simulink model "q_5dof_wand_vr_sphere_collision_atia"  (Simulink 9.1)
settings: Solver=ode1  StartTime=0.0  StopTime=inf  FixedStep=0.001  RelTol=1e-3  EnableMultiTasking=on
values from neighbouring files (symbols this model uses):
  COM = zeros(1,size(V1,2))    [atia_centroid.m]
  fromSI = [1e3 1e3 1e3 180/pi 180/pi]    [setup_wand.m]
  K_CURR = 0.5 * [1 1 -1 -1 1 1]    [setup_wand.m]
  kd = [kd_x kd_y kd_z kd_yaw kd_roll]    [setup_wand.m]
  kp = [kp_x kp_y kp_z kp_yaw kp_roll]    [setup_wand.m]
  vo_c = [0 75 -75] * 1e-3    [setup_wand.m]
  wn_f = 150    [setup_wand.m]
  zeta_f = 1    [setup_wand.m]
undefined symbols (not defined in the file or in its folder): DiscIntNeverNeededParam, HIL, qc_get_step_size, V_CUBE_atia_wand, Visualization
libraries: quarc_library x12
(part 2 of 2)

== matlab function Virtual Cube/Virtual Cube ==
  data: dir_atia output double; center input double; COM input double; V_CUBE_atia_wand input double; k_stiff input double; k_damp input double; w_xyz input double; F output double; w_dot input double; collisionFlag output double; dist output double; F_ATIA output double
% Inputs:
% center    = center of object (m)
% radius    = radius of object (m)
% k_stiff   = Stiffness gain (N/m)
% k_damp    = Damping gain (N.s/m)
% w         = world coordinates of wand (m,rad)
% w_dot     = world rate of wand (m/s,rad/s)
%
% Output: 
% F = Output force (N)
%radius==V_CUBE_atia_wand
function [dir_atia,F,collisionFlag,dist,F_ATIA]  = virtual_object(center,COM,V_CUBE_atia_wand, k_stiff, k_damp, w_xyz, w_dot)
%%%%%%%%%%%%%%%%%%%%%%%%%%%%%%%%%%%%%%%%%%%%%%%%%%%%%%

scale=1;
position=COM;
%[V_CUBE_atia_wand,COM]=atia_shape_vertecise(scale,V_CUBE_atia_wand,center)
% Example script for GJK function
%   Animates two objects on a collision course and terminates animation
%   when they hit each other. Loads vertex and face data from
%   SampleShapeData.m. See the comments of GJK.m for more information
%
%   Most of this script just sets up the animation and transformations of
%   the shapes. The only key line is:
%   collisionFlag = GJK(S1Obj,S2Obj,iterationsAllowed)
%
%   Matthew Sheen, 2016
%
%
%%%%%%%%%%%%%%%%%%%%% MODIFICTATION NOTICE: %%%%%%%%%%%%%%%%%%%%%%%%%%%%%%%
% This script test has been modified and renamed by PHILIPPE LEBEL 
% April 2017
%
% The author of the original script is Matthew Sheen
% published on
% https://www.mathworks.com/matlabcentral/fileexchange/57907-fast-3d-collision-detection-gjk-algorithm
% 
%
%I (Philippe Lebel) modified it to accommodate tests for my implmenetation of GJK distance
%algorithm. The commented section at the end of the code allows to see the
%minkowski difference and the verticies member of the simplex evolving
%durring the simulation.
%
%The function I wrote is [dist,pts,G,H]=GJK_dist(S1Obj,S2Obj);
% I only take credit for this function.
% I also modified some sections of the other matlab files to accommodate my
% new function.
% I want to personnally thank Matthew Sheen for his work. This allowed me
% to understand a lot concerning the implementation of such algorithm.
%
% The algorithm works in the vast majority of cases, but some times, in
% close proximity, the closest distance points are a little off. There is
% work to be done concerning this bug. Feel free to contribute if you find
% something.




%clc;clear all;close all% khodm % krdm

%How many iterations to allow for collision detection.
iterationsAllowed = 6;

% Make a figure
%fig=figure('units','normalized','outerposition',[0 0 1 1]);
%set(fig, 'renderer', 'OpenGL');

% fig = figure;
%hold on

% Load sample vertex and face data for two convex polyhedra
% SampleShapeData;
%[V1,F1]=platonic_solid(1,1);
% I make a cube here with  0.05, and transfer com of that to center of
% yellow cube

%[V_CUBE_atia_wand,F1]=platonic_solid(2,0.05);
%COM=atia_centroid(V_CUBE_atia_wand);
%diff_atia=[0 0 -0.075]-COM;
 %V_CUBE_atia_wand=V_CUBE_atia_wand+diff_atia;
 %COM=atia_centroid(V_CUBE_atia_wand);%cube center
 
%[V2,F2]=platonic_solid(3,1); put a point instead of a tethrahedron
 V2=[0 0 0];
 F2=[1 1 1];
 
% V_CUBE_atia_wand =([ 0.1000  120.0000  -34.9000
 %        0  120.0000  -35.0000
  %  0.1000  120.0000  -35.0000
   %      0  120.0000  -34.9000
    %0.1000  120.1000  -34.9000
     %    0  120.1000  -34.9000
    %0.1000  120.1000  -35.0000
     %    0  120.1000  -35.0000]*0.001)+([0 210 -225]*0.001)+[0 0 0.035];%cube went tp the wand location
 
  V_CUBE_atia=[  100.0000         0  100.0000
         0         0         0
  100.0000         0         0
       0         0  100.0000
100.0000  100.0000  100.0000
        0  100.0000  100.0000
 100.0000  100.0000         0
        0  100.0000         0];
     V_CUBE_atia= V_CUBE_atia*0.001;
% Make shape 1

%coder.extrinsic('patch'); 
%S1.Vertices = V1;
%S1.Faces = F1;
%S1.FaceVertexCData=0;
%S1.FaceVertexCData = jet(size(V1,1));
% S1.FaceColor='white';
%S1.FaceColor = 'interp';
%S1Obj = patch(S1);
%COM=atia_centroid(V1);
%COM=atia_centroid(V_CUBE_atia_wand);
% Make shape 2

%S2.Vertices = V2;% handle nist 
%%S2.FaceVertexCData=0;
%S2.FaceVertexCData = jet(size(V2,1));
% S2.FaceColor='white';
%S2.FaceColor = 'interp';
%S2Obj = patch(S2);%handle

 %atia_void_figure()
%hold off
%axis equal
%axis([-5 5 -5 5 -5 5])
%fig.Children.Visible = 'off'; % Turn off the axis for more pleasant viewing.
%Color=[1 1 1];
%fig.Color = Color;
%rotate3d on;

%S1Obj.Vertices=zeros(20,3);
%S2Obj.Vertices=zeros(1,3);

%Move them through space arbitrarily.
% I have to replace every S1Obj.Vertices with V1
%S1Obj.Vertices=V1;
%S2Obj.Vertices=V2;
%S1Obj=atia_produce_handle(V1,F1);
%S1Coords = S1Obj.Vertices;
%[S2Obj]=atia_produce_handle(V2,F2);
%S2Coords = S2Obj.Vertices;
%S1Coords =V1;
%S2Coords = V2;

%S1Rot = eye(3,3); % Accumulate angle changes

% Make a random rotation matix to rotate shape 1 by every step
%S1Angs = 0.1*rand(3,1); % Euler angles
% S1Angs=[0 0 0.1]';
%sang1 = sin(S1Angs);
%cang1 = cos(S1Angs);
%cx = cang1(1); cy = cang1(2); cz = cang1(3);
%sx = sang1(1); sy = sang1(2);  sz = sang1(3);

%S1RotDiff = ...
 %   [          cy*cz,          cy*sz,            -sy
%    sy*cx*cz+sz*sx, sy*cx*sz-cz*sx,          cy*cx];

%S2Rot = eye(3,3);

% Make a random rotation matix to rotate shape 2 by every step
%S2Angs = 0.1*rand(3,1); % Euler angles
% S2Angs=[0 0 0]';
%sang2 = sin(S2Angs);
%cang2 = cos(S2Angs);
%cx = cang2(1); cy = cang2(2); cz = cang2(3);
%sx = sang2(1); sy = sang2(2); sz = sang2(3);

%S2RotDiff = ...
%    [          cy*cz,          cy*sz,            -sy
%    sy*sx*cz-sz*cx, sy*sx*sz+cz*cx,          cy*sx
%    sy*cx*cz+sz*sx, sy*cx*sz-cz*sx,          cy*cx];

%%%%%%%%%%%%%%%%%%%%%%%%%%%%%%%%%%%%%%%%%%%%%%%%%%%%%%%%%%%%%%%%%%%%%
%%%%%%%%%%%%%%%%%%%%%%%%%%%%%%%%%%%%%%%%%%%%%%%%%%%%%%%%%%%%%%%%%%%%


% Animation loop. Terminates on collision.
%n=1;
%dist=-1000;
%for i = 2:-0.005:-inf;
%     if n==60
%         break
%     end


%    S1Rot = S1RotDiff*S1Rot;
%    S2Rot = S2RotDiff*S2Rot;
    %S2Rot = [0.0580    0.9510    0.3037];
    
    %S1Obj.Vertices = (S1Rot*S1Coords')' ;
    %S2Obj.Vertices=w_xyz;
%    V1 = (S1Rot*S1Coords')' ;
%    V2=(w_xyz)';
    %S2Obj.Vertices = (S2Rot*S2Coords')'+-i;%point w_xyz
  
    %[S,D]=minksum(V1,-V2);
   % stock.s{n}=S;
   % stock.s1{n}=S1Obj;
   % stock.s2{n}=S2Obj;
    % Do collision detection
   %collisionFlag = GJK(V_CUBE_atia_wand,(w_xyz'),iterationsAllowed);
    %collisionFlag = GJK(S1Obj,S2Obj,iterationsAllowed);
    %[dist,pts,G,H] = GJK_dist( V_CUBE_atia_wand, (w_xyz') )
     %collisionFlag = GJK_mod(V_CUBE_atia_wand,(w_xyz)',iterationsAllowed);
  [a,b,c,d,collisionFlag] = GJK_mod(V_CUBE_atia_wand,(w_xyz'),iterationsAllowed);
    
    %coder.extrinsic('tic');
    %[dist,pts,G,H]=GJK_dist(V1,V2);
    [dist,pts,G,H]=GJK_dist(V_CUBE_atia_wand,(w_xyz)');
    radius_atia=norm(G-(COM));%radius of cube
    r_atia=w_xyz-(COM);
    r_abs_atia=norm(r_atia);
    %coder.extrinsic('toc');
%     stock.pts{n}=pts;
    %try delete(hhh)
    %end
    %hold on
    %plot3(G(1),G(2),G(3),'Ob','Linewidth',3);
    %hold on
   % plot3(H(1),H(2),H(3),'Ob','Linewidth',3);
    %hold on
   %line([G(1) H(1)],[G(2) H(2)],[G(3) H(3)]);
%     [a,b, c,dist]=EPA(a,b,c,d);
    %stock.pts{n}=pts;
    %dist_acc(n)=dist;
%     [q,r]=max(abs(diff(dist_acc)))
%     if max(abs(diff(dist_acc)))>0.1
%         break
%     end
    %n=n+1;
    %drawnow;
    %hold on
    %figure
    dir_atia = (r_atia) / norm((r_atia));
    %plot(collisionFlag(n))
    if collisionFlag
     %if (r_abs_atia<=radius_atia) very ineffective
       % t = text(3,3,3,'Collision!','FontSize',30);
       %  break;
          %dir=w_xyz-(COM)';
         %dir_atia = (r_atia) / norm((r_atia));
         %F_stiff = [dir_atia * k_stiff(1)*100000000000000 *(radius_atia-r_abs_atia); 0; 0];
         %10000000000000000000000 
         F_stiff = [dir_atia * k_stiff(1)* dist; 0; 0];
           %F_stiff = [dir * k_stiff(1)*1000 * norm(w_xyz-(COM)'); 0; 0];
            %F_stiff = [dir * k_stiff(1) * collisionFlag ; 0; 0];
            
    %F_stiff = [dir * k_stiff(1) * (radius - norm(r)); 0; 0];% r_abs replaced by norm(r)
    % damping force (N)
    %100000000000000
    F_damp = - k_damp .* w_dot;
    % total force
    F = F_stiff + F_damp;
    % = F_stiff;
    F_ATIA=F(1:3,1) ;  
    else
         %t = text(3,3,3,' No Collision!','FontSize',30);
         F = [ 0; 0; 0; 0; 0 ];
         F_ATIA=F(1:3,1) ;
    %end
     %drawnow;
    end
%hold on
%figure
%plot(w_xyz(n))
%disp('w_xyz(n)')
%hold on
%dist_acc(end)
% figure
% view(3)
% for i=1:3:length(stock.s)
%     a=stock.s{i};
%     pts=stock.pts{i};
%     pt_x=a(:,1);
%     pt_y=a(:,2);
%     pt_z=a(:,3);
%     T = delaunay(pt_x,pt_y,pt_z);
%     X=[pt_x,pt_y,pt_z];
%     try delete(h1)
%     end
%     try delete(h2)
%     end
%     h1=tetramesh(T,X,'faceColor','b','EdgeColor',[0 0 0],'FaceAlpha',0.1);
%     hold on
%     for j=1:3
%         h2(j)=plot3(pts(1,j),pts(2,j),pts(3,j),'Or','LineWidth',3);
%         hold on
%         d=cross(pts(:,2)-pts(:,1),pts(:,3)-pts(:,1));
%         if d'*pts(:,1)>0
%             d=-d;
%         end
%         line([pts(1,1) pts(1,1)+d(1)],[pts(2,1) pts(2,1)+d(2)],[pts(3,1) pts(3,1)+d(3)])
%         hold on
%     end
%     hold off
%     
%     axis([-1 10 -1 10 -1 10]);
%     drawnow;
%     pause(0.05)
% end
% hold on%%%%%%%%%%%%%%%%%%%%%%%%%

% Vector from object to wand (m)
r = w_xyz - center;
% Distance of r (m)
r_abs = norm( r );
% Is wand inside object?
%if ( (norm(r(1)) < radius) && (norm(r(2)) < radius) && (norm(r(3)) < radius)&& (norm(r)>radius)&&(norm(r)<1.73*radius))
%if((r_abs<radius) )  
% normalized direction vector
    dir = r / norm(r); % r_abs replaced by norm(r)   
    % stiffness force (N)
     %F_stiff = [dir * k_stiff(1) * (radius-r_abs); 0; 0];
    %F_stiff = [dir * k_stiff(1) * (radius - norm(r)); 0; 0];% r_abs replaced by norm(r)
    % damping force (N)
   % F_damp = - k_damp .* w_dot;
    % total force
   % F = F_stiff + F_damp ;
%else
    % Want not touching object.
   % F = [ 0; 0; 0; 0; 0 ];
end

function [V_CUBE_atia_wand,COM]=atia_shape_vertecise(scale,V_CUBE_atia_wand,center)
%[V_CUBE_atia_wand,F]=platonic_solid(n,r);
V_CUBE_atia_wand=V_CUBE_atia_wand*scale;
COM=atia_centroid(V_CUBE_atia_wand);
diff_atia=center'-COM;
 V_CUBE_atia_wand=V_CUBE_atia_wand+diff_atia;
 COM=atia_centroid(V_CUBE_atia_wand);%cube center
end

function COM=atia_centroid(V1)%
% this function take a matris V1 as input, find average for each column,
% and give you mean or center of mass
COM=zeros(1,size(V1,2));
for j=1:size(V1,2)
s1=0;
for i=1:size(V1,1)%20-7
  %  s1=s1+ eval(sprintf('V1%d(i,1)',j));% adds up X value for all columns%p-V1
    % s1=s1+ eval(V1(sprintf('%d',i),j));
      s1=s1+ V1(i,j);
end
COM(1,j)=s1/size(V1,1);%20-7
end
end


%This function is based on the book Real-Time Collision Detection
% (http://realtimecollisiondetection.net/)
%
%It computes the distance, the points of closest proximity points and also
%returns the points last contained in the simplex.
%[dist,pts,G,H] = GJK_dist_7_point_poly( shape1, shape2 )
%
% INPUTS:
%
% shape1:   a patch object representing the first convex solid
% shape2:   a patch object representing the second convex solid
%
% OUTPUTS:
%
% dist:     an absolute float number representing the minimum distance between
%           the shapes.
% pts:      The points of the minkowsky diference where the alogrithm
%           stoped.
% G:        The point on shape1 closest to shape2
% H:        The point on shape2 closest to shape1


% updated 05/01/17. Thanks to Amin Ramezanifar for pointing out an error.


function [dist,pts,G,H] = GJK_dist( shape1, shape2 )

%pick a random direction
d=[1 1 1];
%pick a point
[a, point1_a, point2_a]=support_2(shape1,shape2,d);
%pick a second point to creat a line
[b, point1_b, point2_b]=support_2(shape1,shape2,-d);
%pick a third point to make a tirangle
ab=b-a;
ao=-a;
%perpendicular direction
d=cross(cross(ab,ao),ab);
%pick a third point
[c, point1_c, point2_c]=support_2(shape1,shape2,d);
%the simplex is now complete
pts=[a b c];
pts_1_2=[point1_a point1_b point1_c;point2_a point2_b point2_c];


itt=0;
pts_old=pts;
norm_old=norm(pts_old);
d_old=d;
dist_old=1000;
dist=1000;
flag=0;
%PP0 = 'V';
PP0 = [3 4 12];
%This loop is there for the very rare case where the simplex would contain
%duplicate points.
while true
    if isequal(c,b) || isequal(c,a)
        [c, point1_c, point2_c]=support_2(shape1,shape2,-d);
    else
        pts=[a b c];
        pts_1_2=[point1_a point1_b point1_c;point2_a point2_b point2_c];
        break
    end
end
while true
    
    %we compute the norm of vector going from the origin to each member
    %of the simplex
    Norm_pts = (sqrt(sum(abs(pts').^2,2)));
    %Computing and removing the farthest point of the simplex from the origin
    [max_norm,index]=max(Norm_pts);

    %new search direction
    d=cross(pts(:,2)-pts(:,1),pts(:,3)-pts(:,1));
    origin_projected=(pts(:,1)'*d)*d;
    if d'*origin_projected>0
        d=-d;
    end
    d=d/norm(d);
    
    
    %Pciking a new point to add to the simplex.
    [c, point1_c, point2_c]=support_2(shape1,shape2,d);
    %we project the origin on the simplex's plane.
    origin_projected=(pts(:,1)'*d)*d;
    % We verify if the point is allready contained in the simplex.
    % The (itt>5 && flag == 5) condition to enter this loop is one of the main
    % problems of the algorithm. Sometime, when using only the normal to
    % the triangle, the solution does not converge to the absolute minimum
    % distance. This other way of computing the new direction allows a
    % higher rate of succesful convergeance. If one would want to upgrade the
    % algorithm he would certainly need to work arround here.
     if any(abs(Norm_pts-norm(c))<0.000001) || (itt>5 && flag == 5)
         % computing the distance of each traingle lines from the origin
        d1 = distLinSeg(pts(:,1)',pts(:,2)',origin_projected',origin_projected');
        d2 = distLinSeg(pts(:,1)',pts(:,3)',origin_projected',origin_projected');
        d3 = distLinSeg(pts(:,2)',pts(:,3)',origin_projected',origin_projected');
%         d1=(pts(:,2)-pts(:,1))'/norm(pts(:,2)-pts(:,1))*(pts(:,1)-origin_projected)/norm((pts(:,1)-origin_projected));
%         d2=(pts(:,3)-pts(:,1))'/norm(pts(:,3)-pts(:,1))*(pts(:,1)-origin_projected)/norm((pts(:,1)-origin_projected));
%         d3=(pts(:,3)-pts(:,2))'/norm(pts(:,3)-pts(:,2))*(pts(:,2)-origin_projected)/norm((pts(:,2)-origin_projected));
        dist_seg_min=min(abs([d1 d2 d3]));
        %we want to pick the two points creating the line closest to the
        %origin.
        %We also need to deal with the case where the origin is closest to
        %a point, resulting in two distances being equal.
        if dist_seg_min<dist
            while true
                if d1==dist_seg_min
                    %pick a third point to make a tirangle
                    ab=pts(:,2)-pts(:,1);
                    ao=-pts(:,1);
                    %perpendicular direction
                    d=cross(cross(ab,ao),ab);
                    if d1~=d2 && d1~=d3
                        [c, point1_c, point2_c]=support_2(shape1,shape2,d);
                        index=3;
                        break
                    else
                        [c_1, point1_c_1, point2_c_1]=support_2(shape1,shape2,d);
                        index_1=3;
                    end
                end
                if d2==dist_seg_min
                    %pick a third point to make a tirangle
                    ab=pts(:,3)-pts(:,1);
                    ao=-pts(:,1);
                    %perpendicular direction
                    d=cross(cross(ab,ao),ab);
                    if d2~=d1 && d2~=d3
                        [c, point1_c, point2_c]=support_2(shape1,shape2,d);
                        index=2;
                        break
                    else
                        [c_2, point1_c_2, point2_c_2]=support_2(shape1,shape2,d);
                        index_2=2;
                    end
                end
                if d3==dist_seg_min
                    %pick a third point to make a tirangle
                    ab=pts(:,3)-pts(:,2);
                    ao=-pts(:,2);
                    %perpendicular direction
                    d=cross(cross(ab,ao),ab);
                    if d3~=d1 && d3~=d2
                        [c, point1_c, point2_c]=support_2(shape1,shape2,d);
                        index=1;
                        break
                    else
                        [c_3, point1_c_3, point2_c_3]=support_2(shape1,shape2,d);
                        index_3=1;
                    end
                    
                end
                if d1==d2
                    L1=(pts(:,2)-pts(:,1))'/norm(pts(:,2)-pts(:,1))*(pts(:,1)-origin_projected)/norm((pts(:,1)-origin_projected));
                    L2=(pts(:,3)-pts(:,1))'/norm(pts(:,3)-pts(:,1))*(pts(:,1)-origin_projected)/norm((pts(:,1)-origin_projected));
                    if L1>L2%%%%%%%%%%%%%%%% edit c_1
                        
                    ab=pts(:,2)-pts(:,1);
                    ao=-pts(:,1);
                    %perpendicular direction
                    d=cross(cross(ab,ao),ab);
                    [c_1, point1_c_1, point2_c_1]=support_2(shape1,shape2,d);
                        c=c_1;
                        point1_c=point1_c_1;
                        point2_c=point2_c_1;
                    else%%%%%%%%%%%%%%%edit c_2
                                            %pick a third point to make a tirangle
                    ab=pts(:,3)-pts(:,1);
                    ao=-pts(:,1);
                    %perpendicular direction
                    d=cross(cross(ab,ao),ab);
                    [c_2, point1_c_2, point2_c_2]=support_2(shape1,shape2,d);
                        c=c_2;
                        point1_c=point1_c_2;
                        point2_c=point2_c_2;
                    end
                elseif d1==d3
                    L1=(pts(:,2)-pts(:,1))'/norm(pts(:,2)-pts(:,1))*(pts(:,1)-origin_projected)/norm((pts(:,1)-origin_projected));
                    L3=(pts(:,3)-pts(:,2))'/norm(pts(:,3)-pts(:,2))*(pts(:,2)-origin_projected)/norm((pts(:,2)-origin_projected));
                    if L1>L3
                                            ab=pts(:,2)-pts(:,1);
                    ao=-pts(:,1);
                    %perpendicular direction
                    d=cross(cross(ab,ao),ab);
                     [c_1, point1_c_1, point2_c_1]=support_2(shape1,shape2,d);
                        c=c_1;
                        point1_c=point1_c_1;
                        point2_c=point2_c_1;
                    else%%%%%%%%%%%%%%% edit c_3
                                            ab=pts(:,3)-pts(:,2);
                    ao=-pts(:,2);
                    %perpendicular direction
                    d=cross(cross(ab,ao),ab);
                    [c_3, point1_c_3, point2_c_3]=support_2(shape1,shape2,d);
                        c=c_3;
                        point1_c=point1_c_3;
                        point2_c=point2_c_3;
                    end
                elseif d2==d3
                    L2=(pts(:,3)-pts(:,1))'/norm(pts(:,3)-pts(:,1))*(pts(:,1)-origin_projected)/norm((pts(:,1)-origin_projected));
                    L3=(pts(:,3)-pts(:,2))'/norm(pts(:,3)-pts(:,2))*(pts(:,2)-origin_projected)/norm((pts(:,2)-origin_projected));
                    if L2>L3%%%%%%%%%%%%%%% editc_2
                                            ab=pts(:,3)-pts(:,1);
                    ao=-pts(:,1);
                    %perpendicular direction
                    d=cross(cross(ab,ao),ab);
                    [c_2, point1_c_2, point2_c_2]=support_2(shape1,shape2,d);
                        c=c_2;
                        point1_c=point1_c_2;
                        point2_c=point2_c_2;
                    else%%%%%%%%%%%% edit c_3
                          [c_3, point1_c_3, point2_c_3]=support_2(shape1,shape2,d);
                        index_3=1;
                        c=c_3;
                        point1_c=point1_c_3;
                        point2_c=point2_c_3;
                    end
                end
                break
            end
        end
        % if even after picking a new point with the other method, if the
        % simplex already has it, we assume we converged.
        if any(abs(Norm_pts-norm(c))<0.000001)
            if (norm(PP0) == 13)
                % converged on first itteration, dist and PP0 must be
                % computed.
                [dist, PP0] = pointTriangleDistance(pts',[0 0 0]);
            end
            Norm_pts=0;
            break
        end
     end
    
    %pts(:,index)=[];
    atia_index=zeros(3,2);%%% this functionn is allocated instead of pts(:,index)=[];
       if (index==1)
            atia_index=pts(:,[2,3]);
            %atia_index=pts(:,(size(pts,2)-index):size(pts,2));% instead of deleting a column, I define atia
           %pts=[atia_index c];
       elseif (index==2)
                     atia_index=pts(:,[1,3]);
                     %atia_index=pts(:,(size(pts,2)-index):2:size(pts,2));
       else
                     atia_index=pts(:,[1,2]);
                    %atia_index=pts(:,1:(size(pts,2)-1):size(pts,2));
       end
   
    pts=[atia_index c];

    %pts_1_2(:,index)=[];
    
       % switch index %this switch is replaced by :pts_1_2(:,index)=[];
    %case 1
     %   atia_index_pts_1_2=pts_1_2(:,[2,3]);
    %case 2
     %   atia_index_pts_1_2=pts_1_2(:,[1,3]);
    %case 3
     %   atia_index_pts_1_2=pts_1_2(:,[1,2]);
      %  end
      if (index==1)
          atia_index_pts_1_2=pts_1_2(:,[2,3]);
      elseif (index==2)
          atia_index_pts_1_2=pts_1_2(:,[1,3]);
      else
          atia_index_pts_1_2=pts_1_2(:,[1,2]);
      end
    
    
    %pts=[pts c];
    pts_1_2=[atia_index_pts_1_2 [point1_c;point2_c]];
    %pts_1_2=[pts_1_2 [point1_c;point2_c]];
    [dist, PP0] = pointTriangleDistance(pts',[0 0 0]);
    %we need to do the following manipulation because sometimes, the
    %simplex will oscillate arround the closest solution, creating an
    %infinite loop. We need to backup the solution that resulted in the
    %minimal distance and use it if the loop times out (10 itteration max)
    if dist<dist_old
        pts_prox=pts;
        dist_prox=dist;
        PP0_prox=PP0;
        pts_1_2_prox=pts_1_2;
    end
    
    %The time out is set here.
    if itt>6
        flag=5;
        if itt>10 && flag==5
            pts_prox=pts;%%edit 582, proxy pts
            pts=pts_prox;
            dist_prox=dist;%%% 584 edit
            dist=dist_prox;
            PP0_prox=PP0;%%% 586 edit
            PP0=PP0_prox;
            pts_1_2_prox=pts_1_2;%%% edit 588
            pts_1_2=pts_1_2_prox;
            break
        end
        
    end

    dist_old=dist;
    d_old=d;
    pts_old=pts;
    if abs(norm_old-norm(pts))<0.01
        norm_old=norm(pts);
    end
    itt=itt+1;
    
%         pause(0.1)
end

% Calculation of the barycentric coordinates of the origin in respect to
% the simplex.
 T = [1	 4  3;
      1  4  2;
      3	 4  2;
      1  2  3];
  pts_t=[pts';PP0];
  coder.extrinsic('triangulation');
  %TR=zeros(4,3);
  %TR=triangulation(T,pts_t);
  %coder.extrinsic('cartesianToBarycentric');
  %B=[0 0 0];
  %B=cartesianToBarycentric(TR,4,PP0);
   B = [pts_t(4,:),1]/[pts_t(1:3,:),ones(3,1)];% solution instead of "triangulation" and "cartesianToBarycentric"
  G=[0 ;0; 0];
  H=[0 ;0 ;0];
  %calculation of the points G and H of proximity on,respectively, shape1
  %and shape2.
  for i=1:3
      G=G+B(i)*pts_1_2(1:3,i);
      H=H+B(i)*pts_1_2(4:6,i);
  end
end























function [flag] = GJK(shape1,shape2,iterations)
% GJK Gilbert-Johnson-Keerthi Collision detection implementation.
% Returns whether two convex shapes are are penetrating or not
% (true/false). Only works for CONVEX shapes.
%
% Inputs:
%   shape1: 
%   must have fields for XData,YData,ZData, which are the x,y,z 
%   coordinates of the vertices. Can be the same as what comes out of a 
%   PATCH object. It isn't required that the points form faces like patch
%   data. This algorithm will assume the convex hull of the x,y,z points
%   given.
%
%   shape2: 
%   Other shape to test collision against. Same info as shape1.
%   
%   iterations: 
%   The algorithm tries to construct a tetrahedron encompassing
%   the origin. This proves the objects have collided. If we fail within a
%   certain number of iterations, we give up and say the objects are not
%   penetrating. Low iterations means a higher chance of false-NEGATIVES
%   but faster computation. As the objects penetrate more, it takes fewer
%   iterations anyway, so low iterations is not a huge disadvantage.
%   
% Outputs:
%   flag:
%   true - objects collided
%   false - objects not collided
%
%  
%   This video helped me a lot when making this: https://mollyrocket.com/849
%   Not my video, but very useful.
%   
%   Matthew Sheen, 2016
%

%Point 1 and 2 selection (line segment)
v = [0.8 0.5 1];
[a,b] = pickLine(v,shape2,shape1);

%Point 3 selection (triangle)
[a,b,c,flag] = pickTriangle(a,b,shape2,shape1,iterations);
%Point 4 selection (tetrahedron)
if flag == 1 %Only bother if we could find a viable triangle.
    [a,b,c,d,flag] = pickTetrahedron(a,b,c,shape2,shape1,iterations);
end

end

function [a,b] = pickLine(v,shape1,shape2)
%Construct the first line of the simplex
b = support(shape2,shape1,v);
a = support(shape2,shape1,-v);
end

function [a,b,c,flag] = pickTriangle(a,b,shape1,shape2,IterationAllowed)
flag = 0; %So far, we don't have a successful triangle.

%First try:
ab = b-a;
ao = -a;
v = cross(cross(ab,ao),ab); % v is perpendicular to ab pointing in the general direction of the origin.

c = b;
b = a;
a = support(shape2,shape1,v);

for i = 1:IterationAllowed %iterations to see if we can draw a good triangle.
    %Time to check if we got it:
    ab = b-a;
    ao = -a;
    ac = c-a;
    
    %Normal to face of triangle
    abc = cross(ab,ac);
    
    %Perpendicular to AB going away from triangle
    abp = cross(ab,abc);
    %Perpendicular to AC going away from triangle
    acp = cross(abc,ac);
    
    %First, make sure our triangle "contains" the origin in a 2d projection
    %sense.
    %Is origin above (outside) AB?   
    if dot(abp,ao) > 0
        c = b; %Throw away the furthest point and grab a new one in the right direction
        b = a;
        v = abp; %cross(cross(ab,ao),ab);
        
        %Is origin above (outside) AC?
    elseif dot(acp, ao) > 0
        b = a;
        v = acp; %cross(cross(ac,ao),ac);
        
    else
        flag = 1;
        break; %We got a good one.
    end
    a = support(shape2,shape1,v);
end
end

function [a,b,c,d,flag] = pickTetrahedron(a,b,c,shape1,shape2,IterationAllowed)
%Now, if we're here, we have a successful 2D simplex, and we need to check
%if the origin is inside a successful 3D simplex.
%So, is the origin above or below the triangle?
flag = 0;

ab = b-a;
ac = c-a;

%Normal to face of triangle
abc = cross(ab,ac);
ao = -a;

if dot(abc, ao) > 0 %Above
    d = c;
    c = b;
    b = a;
    
    v = abc;
    a = support(shape2,shape1,v); %Tetrahedron new point
    
else %below
    d = b;
    b = a;
    v = -abc;
    a = support(shape2,shape1,v); %Tetrahedron new point
end

for i = 1:IterationAllowed %Allowing 10 tries to make a good tetrahedron.
    %Check the tetrahedron:
    ab = b-a;
    ao = -a;
    ac = c-a;
    ad = d-a;
    
    %We KNOW that the origin is not under the base of the tetrahedron based on
    %the way we picked a. So we need to check faces ABC, ABD, and ACD.
    
    %Normal to face of triangle
    abc = cross(ab,ac);
    
    if dot(abc, ao) > 0 %Above triangle ABC
        %No need to change anything, we'll just iterate again with this face as
        %default.
    else
        acd = cross(ac,ad);%Normal to face of triangle
        
        if dot(acd, ao) > 0 %Above triangle ACD
            %Make this the new base triangle.
            b = c;
            c = d;
            ab = ac;
            ac = ad;            
            abc = acd;     
        elseif dot(acd, ao) < 0
            adb = cross(ad,ab);%Normal to face of triangle
            
            if dot(adb, ao) > 0 %Above triangle ADB
                %Make this the new base triangle.
                c = b;
                b = d;              
                ac = ab;
                ab = ad;
                abc = adb;           
            else
                flag = 1; 
                break; %It's inside the tetrahedron.
            end
        else %the origin is on the same plane as the triangle
            ;
        end
    end
    
    %try again:
    if dot(abc, ao) > 0 %Above
        d = c;
        c = b;
        b = a;    
        v = abc;
        a = support(shape2,shape1,v); %Tetrahedron new point
    else %below
        d = b;
        b = a;
        v = -abc;
        a = support(shape2,shape1,v); %Tetrahedron new point
    end
end

end

function point = getFarthestInDir(shape, v)
%Find the furthest point in a given direction for a shape
XData = shape(:,1); % Making it more compatible with previous MATLAB releases.
YData = shape(:,2);
ZData = shape(:,3);
dotted = XData*v(1) + YData*v(2) + ZData*v(3);
[maxInCol,rowIdxSet] = max(dotted);
[maxInRow,colIdx] = max(maxInCol);
rowIdx = rowIdxSet(colIdx);
point = [XData(rowIdx,colIdx), YData(rowIdx,colIdx), ZData(rowIdx,colIdx)]';
end

function point = support(shape1,shape2,v)
%Support function to get the Minkowski difference.
point1 = getFarthestInDir(shape1, v);
point2 = getFarthestInDir(shape2, -v);
point = point1 - point2;
end


%function [SObj]=atia_produce_handle(V,F)%thias function produces patch,

%S1.Vertices = V;
%S1.Faces = F;
%S1.FaceVertexCData=0;
%coder.extrinsic('jet'); 
%S1.FaceVertexCData = jet(size(V,1));
% S1.FaceColor='white';
%S1.FaceColor = 'interp';
%coder.extrinsic('patch'); 
%SObj = patch(S1);
%SObj.vertices=S1.Vertices;
%end

function atia_void_figure()
hold off
axis equal
axis([-5 5 -5 5 -5 5])
fig.Children.Visible = 'off'; % Turn off the axis for more pleasant viewing.
Color=[1 1 1];
fig.Color = Color;
rotate3d on;

end


function [V,F]=platonic_solid(n,r)


% ------------------------------------------------------------------------
% PLATONIC_SOLID Creates the PATCH data, the vertices (V) and faces (F) for
% a given platonic solid (according to "n" see below) with radius (r)
%
% n=1 -> Tetrahedron
% n=2 -> Cube
% n=3 -> Octahedron
% n=4 -> Icosahedron
% n=5 -> Dodecahedron
%
% %%%Example
% clear all; close all; clc;
% 
% r=1;
% figure;fig=gcf; clf(fig); colordef (fig, 'white'); units=get(fig,'units'); set(fig,'units','normalized','outerposition',[0 0 1 1]); set(fig,'units',units); set(fig,'Color',[1 1 1]);
% hold on; 
% 
% [V,F]=platonic_solid(1,r);
% subplot(2,3,1);
% patch('Faces',F,'Vertices',V,'FaceColor','b','FaceAlpha',0.6,'EdgeColor','k','LineWidth',2); axis equal; grid on; hold on; view(3); axis off;
% 
% [V,F]=platonic_solid(2,r);
% subplot(2,3,2);
% patch('Faces',F,'Vertices',V,'FaceColor','b','FaceAlpha',0.6,'EdgeColor','k','LineWidth',2); axis equal; grid on; hold on; view(3); axis off;
% 
% [V,F]=platonic_solid(3,r);
% subplot(2,3,3);
% patch('Faces',F,'Vertices',V,'FaceColor','b','FaceAlpha',0.6,'EdgeColor','k','LineWidth',2); axis equal; grid on; hold on; view(3); axis off;
% 
% [V,F]=platonic_solid(4,r);
% subplot(2,3,4);
% patch('Faces',F,'Vertices',V,'FaceColor','b','FaceAlpha',0.6,'EdgeColor','k','LineWidth',2); axis equal; grid on; hold on; view(3); axis off;
% 
% [V,F]=platonic_solid(5,r);
% subplot(2,3,5);
% patch('Faces',F,'Vertices',V,'FaceColor','b','FaceAlpha',0.6,'EdgeColor','k','LineWidth',2); axis equal; grid on; hold on; view(3); axis off;
%
%
% Kevin Mattheus Moerman
% kevinmoerman@hotmail.com
% 13/11/2009
% ------------------------------------------------------------------------

phi=(1+sqrt(5))/2;

switch n
    case 1 % Tetrahedron
        V1=[-0.5;0.5;0;0;];
        V2=[-sqrt(3)/6;  -sqrt(3)/6; sqrt(3)/3; 0];
        V3=[-0.25.*sqrt(2/3); -0.25.*sqrt(2/3); -0.25.*sqrt(2/3);  0.75.*sqrt(2/3)];
        F= [1 2 3; 1 2 4; 2 3 4; 1 3 4;];

    case 2 % Cube
        V1=[-1;  1; 1; -1; -1;  1; 1; -1;];
        V2=[-1; -1; 1;  1; -1; -1; 1;  1;];
        V3=[-1; -1;-1; -1;  1;  1; 1;  1;];
        F= [1 2 3 4; 1 2 6 5; 2 3 7 6; 3 4 8 7; 4 1 5 8; 5 6 7 8;];

    case 3 % Octahedron
        V1=[-1;  1; 1; -1;  0;   0;];
        V2=[-1; -1; 1;  1;  0;   0;];
        V3=[ 0;   0; 0;  0; -1;  1;];
        F= [1 2 5; 2 3 5; 3 4 5; 4 1 5; 1 2 6; 2 3 6; 3 4 6; 4 1 6;];

    case 4 % Icosahedron
        V1=[0;0;0;0;-1;-1;1;1;-phi;phi;phi;-phi;];
        V2=[-1;-1;1;1;-phi;phi;phi;-phi;0;0;0;0;];
        V3=[-phi;phi;phi;-phi;0;0;0;0;-1;-1;1;1;];
        F= [1 4 9;1 5 9;1 8 5;1 8 10;1 10 4; 12 2 5; 12 2 3; 12 3 6; 12 6 9; 12 9 5; 11 7 10; 11 10 8; 11 8 2; 11 2 3; 11 3 7; 2 5 8; 10 4 7; 3 6 7; 6 7 4; 6 4 9; ];

    case 5 % Dodecahedron
        V1=[1;(1/phi);-phi;phi;-1;0;-phi;1;-1;-1;1;(1/phi);-1;0;0;-(1/phi);phi;-(1/phi);1;0;];
        V2=[1;0;-(1/phi);(1/phi);1;-phi;(1/phi);-1;1;-1;-1;0;-1;-phi;phi;0;-(1/phi);0;1;phi;];
        V3=[[1;phi;0;0;-1;-(1/phi);0;1;1;1;-1;-phi;-1;(1/phi);-(1/phi);phi;0;-phi;-1;(1/phi);]];
        F=[1,2,16,9,20;2,16,10,14,8;16,9,7,3,10;7 9 20 15 5;5,7,3,13,18;3,13,6,14,10;6,13,18,12,11;6,11,17,8,14;11,12,19,4,17;1,2,8,17,4;1,4,19,15,20;12,18,5,15,19];

    otherwise
        warning('False input for n')
end

[THETA,PHI,R]=cart2sph(V1,V2,V3);
R=r.*ones(size(V1(:,1)));
[V1,V2,V3]=sph2cart(THETA,PHI,R);
V=[V1 V2 V3];
end







function [S,D]=minksum(A,B)
% MINKSUM Minkowski sum of two arrays
%   S=MINKSUM(A,B) produces the Minkowski sum of two sets A and B
%   in Euclidean space, the result being the addition of every element
%   of A to every element of B.
%
%   [S,D]=MINKSUM(A,B) returns the Minkowski sum S, and also the
%   multiplicity of each element in S.
%
%   The number of columns represent the dimensionality. An array of M points
%   in N-D space is an MxN array. A vector of 1D values is a column vector.
%
%   If the sizes of A and B are MAxN and MBxN respectively, then the size
%   of S will be at most (MA*MB)xN
% 
%   Example:
%     A=[1 1; 2 1; 2 2; 1 2]; B=[3 3; 4 3; 4 4; 3 4];
%     [S,D]=minksum(A,B);
%     plot(A(:,1),A(:,2),'*',B(:,1),B(:,2),'s',S(:,1),S(:,2),'d')
%     axis([0 7 0 7])
%

%   Mike Sheppard
%   Last Modified: 7-Dec-2011


if nargin<2
    error('Requires two inputs');
end
szA=size(A); szB=size(B);
if (szA(2)~=szB(2)) || numel(szA)>2 || numel(szB)>2
    error('Input arrays must be MxN arrays, with equal N');
end

%Pre-allocate memory
S=zeros(szA(1)*szB(1),szA(2));

%Loop through each dimension
for k=1:szA(2)
   temp=bsxfun(@plus,A(:,k),B(:,k)');
   S(:,k)=temp(:);
end

%Take unique for each row
[S,I,J]=unique(S,'rows');
D=histc(J,1:length(I));

end








function [a,b,c,d,flag] = GJK_mod(shape1,shape2,iterations)
% GJK Gilbert-Johnson-Keerthi Collision detection implementation.
% Returns whether two convex shapes are are penetrating or not
% (true/false). Only works for CONVEX shapes.
%
% Inputs:
%   shape1: 
%   must have fields for XData,YData,ZData, which are the x,y,z 
%   coordinates of the vertices. Can be the same as what comes out of a 
%   PATCH object. It isn't required that the points form faces like patch
%   data. This algorithm will assume the convex hull of the x,y,z points
%   given.
%
%   shape2: 
%   Other shape to test collision against. Same info as shape1.
%   
%   iterations: 
%   The algorithm tries to construct a tetrahedron encompassing
%   the origin. This proves the objects have collided. If we fail within a
%   certain number of iterations, we give up and say the objects are not
%   penetrating. Low iterations means a higher chance of false-NEGATIVES
%   but faster computation. As the objects penetrate more, it takes fewer
%   iterations anyway, so low iterations is not a huge disadvantage.
%   
% Outputs:
%   flag:
%   true - objects collided
%   false - objects not collided
%   [a,b,c,d] - members of the simplex
%
%  
%   This video helped me a lot when making this: https://mollyrocket.com/849
%   Not my video, but very useful.
%   
%   Matthew Sheen, 2016
%
%   Modified:
%   Philippe Lebel, 2016:
%   Fixed a bug where aligned vertices would trigger the collision flag
%   while there was no collision ( line 191 )

%Point 1 and 2 selection (line segment)
v = [0.8 0.5 1];
[a,b] = pickLine(v,shape2,shape1);

%Point 3 selection (triangle)
[a,b,c,flag] = pickTriangle(a,b,shape2,shape1,iterations);
%Point 4 selection (tetrahedron)
% if flag == 1 %Only bother if we could find a viable triangle.
    [a,b,c,d,flag] = pickTetrahedron(a,b,c,shape2,shape1,iterations);
% end

end

%%%%%%%%%%%%%%%%%%%%%%%%%%%%%%%%%%%
%function [a,b] = pickLine(v,shape1,shape2)
%Construct the first line of the simplex
%b = support(shape2,shape1,v);
%dir_ori=-b;
%a = support(shape2,shape1,dir_ori);
%nd

%function [a,b,c,flag] = pickTriangle(a,b,shape1,shape2,IterationAllowed)
%flag = 0; %So far, we don't have a successful triangle.

%First try:
%ab = b-a;
%ao = -a;

%v = cross(cross(ab,ao),ab); % v is perpendicular to ab pointing in the general direction of the origin.

%c = b;
%b = a;
%a = support(shape2,shape1,v);

%for i = 1:IterationAllowed %iterations to see if we can draw a good triangle.
    %Time to check if we got it:
 %   ab = b-a;
  %  ao = -a;
   % ac = c-a;
    
    %Normal to face of triangle
 %   abc = cross(ab,ac);
    
    %Perpendicular to AB going away from triangle
%    abp = cross(ab,abc);
    %Perpendicular to AC going away from triangle
%    acp = cross(abc,ac);
    
    %First, make sure our triangle "contains" the origin in a 2d projection
    %sense.
    %Is origin above (outside) AB?   
  %  if dot(abp,ao) > 0
  %      c = b; %Throw away the furthest point and grab a new one in the right direction
  %      b = a;
  %      v = abp; %cross(cross(ab,ao),ab);
        
        %Is origin above (outside) AC?
  %  elseif dot(acp, ao) > 0
 %       b = a;
  %      v = acp; %cross(cross(ac,ao),ac);
        
 %   else
%         flag = 1;
%         break; %We got a good one.
%    end
%    a = support(shape2,shape1,v);
%end
%end
%%%%%%%%%%%%%%%%%%%%%%%%%%%%%%%%%%%%%%%%


%%%%%%%%%%%%%%%%%%%%%%
%function [a,b,c,d,flag] = pickTetrahedron(a,b,c,shape1,shape2,IterationAllowed)
%Now, if we're here, we have a successful 2D simplex, and we need to check
%if the origin is inside a successful 3D simplex.
%So, is the origin above or below the triangle?
%flag = 0;

%ab = b-a;
%ac = c-a;

%Normal to face of triangle
%abc = cross(ab,ac);
%ao = -a;

%if dot(abc, ao) > 0 %Above
%    d = c;
 %   c = b;
 %   b = a;
    
%    v = abc;
%    a_new = support(shape2,shape1,v); %Tetrahedron new point
 %   if ismember(a_new',[a;b;c;d]')
 %   else
 %       d = c;
  %      c = b;
  %      b = a;    
 %       a=a_new;
 %   end
    
%else %below
 %   d = b;
%    b = a;
  %  v = -abc;
 %   a_new = support(shape2,shape1,v); %Tetrahedron new point
 %   if ismember(a_new',[a;b;c;d]')
 %   else
 %       d = b;
 %       b = a;    
 %       a=a_new;
 %   end
%end

%for i = 1:IterationAllowed %Allowing 10 tries to make a good tetrahedron.
    %Check the tetrahedron:
%    ab = b-a;
 %   ao = -a;
 %   ac = c-a;
 %   ad = d-a;
    
    %We KNOW that the origin is not under the base of the tetrahedron based on
    %the way we picked a. So we need to check faces ABC, ABD, and ACD.
    
    %Normal to face of triangle
 %   abc = cross(ab,ac);
    
 %   if dot(abc, ao) > 0 %Above triangle ABC
        %No need to change anything, we'll just iterate again with this face as
        %default.
 %   else
  %      acd = cross(ac,ad);%Normal to face of triangle
        
 %       if dot(acd, ao) > 0 %Above triangle ACD
            %Make this the new base triangle.
  %          b = c;
   %         c = d;
  %          ab = ac;
   %         ac = ad;            
    %        abc = acd;     
    %    elseif dot(acd, ao) < 0
    %        adb = cross(ad,ab);%Normal to face of triangle
            
    %        if dot(adb, ao) > 0 %Above triangle ADB
                %Make this the new base triangle.
    %            c = b;
     %           b = d;              
     %           ac = ab;
     %           ab = ad;
     %           abc = adb;           
     %       else
     %           flag = 1; 
     %           break; %It's inside the tetrahedron.
     %       end
     %   else %The nearest point is one of the three points contained in the simplex
     %       ;
     %   end
   % end
    
    %try again:
   % if dot(abc, ao) > 0 %Above
        
    %    v = abc;
    %    a_new = support(shape2,shape1,v); %Tetrahedron new point
    %    if ismember(a_new',[a;b;c;d]')
    %    else
    %        d = c;
    %        c = b;
    %        b = a;    
     %       a=a_new;
    %    end
        
  %  else %below
        
    %    v = -abc;
    %    a_new = support(shape2,shape1,v); %Tetrahedron new point
    %    if ismember(a_new',[a;b;c;d]')
    %    else
   %         d = b;
   %         b = a;
   %         a=a_new;
  %      end
  %  end
%end

%end
%%%%%%%%%%%%%%%%%%%%%


%%%%%%%%%%%%%%%%%%%%%%%%%%%%%%%%%%%%%$%%
%function point = getFarthestInDir(shape, v)
%Find the furthest point in a given direction for a shape
%XData = shape(:,1); % Making it more compatible with previous MATLAB releases.
%YData = shape(:,2);
%ZData = shape(:,3);
%dotted = XData*v(1) + YData*v(2) + ZData*v(3);
%[maxInCol,rowIdxSet] = max(dotted);
%[maxInRow,colIdx] = max(maxInCol);
%rowIdx = rowIdxSet(colIdx);
%point = [XData(rowIdx,colIdx), YData(rowIdx,colIdx), ZData(rowIdx,colIdx)]';
%end
%%%%%%%%%%%%%%%%%%%%%%%%%%%%%%%%%%%%%%%%

%%%%%%%%%%%%%%%%%%%%%%%
%function point = support(shape1,shape2,v)
%Support function to get the Minkowski difference.
%point1 = getFarthestInDir(shape1, v);
%point2 = getFarthestInDir(shape2, -v);
%point = point1 - point2;
%end
%%%%%%%%%%%%%%%%%%%%%









%This function is based on the book Real-Time Collision Detection
% (http://realtimecollisiondetection.net/)
%
%It computes the distance, the points of closest proximity points and also
%returns the points last contained in the simplex.
%[dist,pts,G,H] = GJK_dist_7_point_poly( shape1, shape2 )
%
% INPUTS:
%
% shape1:   a patch object representing the first convex solid
% shape2:   a patch object representing the second convex solid
%
% OUTPUTS:
%
% dist:     an absolute float number representing the minimum distance between
%           the shapes.
% pts:      The points of the minkowsky diference where the alogrithm
%           stoped.
% G:        The point on shape1 closest to shape2
% H:        The point on shape2 closest to shape1


% updated 05/01/17. Thanks to Amin Ramezanifar for pointing out an error.




function [point,point1 ,point2] = support_2(shape1,shape2,v)% I change all of shape.vertices to only shape
%Support function to get the Minkowski difference.
if size(shape1,1)==1
    point1=shape1(1,:)';
else
    point1 = getFarthestInDir(shape1, v);
end
if size(shape2,1)==1
    point2=shape2(1,:)';
else
    point2 = getFarthestInDir(shape2, -v);
end
point = point1 - point2;
end


function [dist,PP0] = pointTriangleDistance(TRI,P)
% calculate distance between a point and a triangle in 3D
% SYNTAX
%   dist = pointTriangleDistance(TRI,P)
%   [dist,PP0] = pointTriangleDistance(TRI,P)
%
% DESCRIPTION
%   Calculate the distance of a given point P from a triangle TRI.
%   Point P is a row vector of the form 1x3. The triangle is a matrix
%   formed by three rows of points TRI = [P1;P2;P3] each of size 1x3.
%   dist = pointTriangleDistance(TRI,P) returns the distance of the point P
%   to the triangle TRI.
%   [dist,PP0] = pointTriangleDistance(TRI,P) additionally returns the
%   closest point PP0 to P on the triangle TRI.
%
% Author: Gwendolyn Fischer
% Release: 1.0
% Release date: 09/02/02
% Release: 1.1 Fixed Bug because of normalization
% Release: 1.2 Fixed Bug because of typo in region 5 20101013
% Release: 1.3 Fixed Bug because of typo in region 2 20101014

% Possible extention could be a version tailored not to return the distance
% and additionally the closest point, but instead return only the closest
% point. Could lead to a small speed gain.

% Example:
% %% The Problem
% P0 = [0.5 -0.3 0.5];
% 
% P1 = [0 -1 0];
% P2 = [1  0 0];
% P3 = [0  0 0];
% 
% vertices = [P1; P2; P3];
% faces = [1 2 3];
% 
% %% The Engine
% [dist,PP0] = pointTriangleDistance([P1;P2;P3],P0);
% 
% %% Visualization
% [x,y,z] = sphere(20);
% x = dist*x+P0(1);
% y = dist*y+P0(2);
% z = dist*z+P0(3);
% 
% figure
% hold all
% patch('Vertices',vertices,'Faces',faces,'FaceColor','r','FaceAlpha',0.8);
% plot3(P0(1),P0(2),P0(3),'b*');
% plot3(PP0(1),PP0(2),PP0(3),'*g')
% surf(x,y,z,'FaceColor','b','FaceAlpha',0.3)
% view(3)

% The algorithm is based on 
% "David Eberly, 'Distance Between Point and Triangle in 3D',
% Geometric Tools, LLC, (1999)"
% http:\\www.geometrictools.com/Documentation/DistancePoint3Triangle3.pdf
%
%        ^t
%  \     |
%   \reg2|
%    \   |
%     \  |
%      \ |
%       \|
%        *P2
%        |\
%        | \
%  reg3  |  \ reg1
%        |   \
%        |reg0\ 
%        |     \ 
%        |      \ P1
% -------*-------*------->s
%        |P0      \ 
%  reg4  | reg5    \ reg6


%% Do some error checking
if nargin<2
  error('pointTriangleDistance: too few arguments see help.');
end
P = P(:)';
if size(P,2)~=3
  error('pointTriangleDistance: P needs to be of length 3.');
end

if size(TRI)~=[3 3]
  error('pointTriangleDistance: TRI needs to be of size 3x3.');
end

% ToDo: check for colinearity and/or too small triangles.


% rewrite triangle in normal form
B = TRI(1,:);
E0 = TRI(2,:)-B;
%E0 = E0/sqrt(sum(E0.^2)); %normalize vector
E1 = TRI(3,:)-B;
%E1 = E1/sqrt(sum(E1.^2)); %normalize vector


D = B - P;
a = dot(E0,E0);
b = dot(E0,E1);
c = dot(E1,E1);
d = dot(E0,D);
e = dot(E1,D);
f = dot(D,D);

det = a*c - b*b; % do we have to use abs here?
s   = b*e - c*d;
t   = b*d - a*e;

% Terible tree of conditionals to determine in which region of the diagram
% shown above the projection of the point into the triangle-plane lies.
if (s+t) <= det
  if s < 0
    if t < 0
      %region4
      if (d < 0)
        t = 0;
        if (-d >= a)
          s = 1;
          sqrDistance = a + 2*d + f;
        else
          s = -d/a;
          sqrDistance = d*s + f;
        end
      else
        s = 0;
        if (e >= 0)
          t = 0;
          sqrDistance = f;
        else
          if (-e >= c)
            t = 1;
            sqrDistance = c + 2*e + f;
          else
            t = -e/c;
            sqrDistance = e*t + f;
          end
        end
      end %of region 4
    else
      % region 3
      s = 0;
      if e >= 0
        t = 0;
        sqrDistance = f;
      else
        if -e >= c
          t = 1;
          sqrDistance = c + 2*e +f;
        else
          t = -e/c;
          sqrDistance = e*t + f;
        end
      end
    end %of region 3 
  else
    if t < 0
      % region 5
      t = 0;
      if d >= 0
        s = 0;
        sqrDistance = f;
      else
        if -d >= a
          s = 1;
          sqrDistance = a + 2*d + f;% GF 20101013 fixed typo d*s ->2*d
        else
          s = -d/a;
          sqrDistance = d*s + f;
        end
      end
    else
      % region 0
      invDet = 1/det;
      s = s*invDet;
      t = t*invDet;
      sqrDistance = s*(a*s + b*t + 2*d) ...
                  + t*(b*s + c*t + 2*e) + f;
    end
  end
else
  if s < 0
    % region 2
    tmp0 = b + d;
    tmp1 = c + e;
    if tmp1 > tmp0 % minimum on edge s+t=1
      numer = tmp1 - tmp0;
      denom = a - 2*b + c;
      if numer >= denom
        s = 1;
        t = 0;
        sqrDistance = a + 2*d + f; % GF 20101014 fixed typo 2*b -> 2*d
      else
        s = numer/denom;
        t = 1-s;
        sqrDistance = s*(a*s + b*t + 2*d) ...
                    + t*(b*s + c*t + 2*e) + f;
      end
    else          % minimum on edge s=0
      s = 0;
      if tmp1 <= 0
        t = 1;
        sqrDistance = c + 2*e + f;
      else
        if e >= 0
          t = 0;
          sqrDistance = f;
        else
          t = -e/c;
          sqrDistance = e*t + f;
        end
      end
    end %of region 2
  else
    if t < 0
      %region6 
      tmp0 = b + e;
      tmp1 = a + d;
      if (tmp1 > tmp0)
        numer = tmp1 - tmp0;
        denom = a-2*b+c;
        if (numer >= denom)
          t = 1;
          s = 0;
          sqrDistance = c + 2*e + f;
        else
          t = numer/denom;
          s = 1 - t;
          sqrDistance = s*(a*s + b*t + 2*d) ...
                      + t*(b*s + c*t + 2*e) + f;
        end
      else  
        t = 0;
        if (tmp1 <= 0)
            s = 1;
            sqrDistance = a + 2*d + f;
        else
          if (d >= 0)
              s = 0;
              sqrDistance = f;
          else
              s = -d/a;
              sqrDistance = d*s + f;
          end
        end
      end
      %end region 6
    else
      % region 1
      numer = c + e - b - d;
      if numer <= 0
        s = 0;
        t = 1;
        sqrDistance = c + 2*e + f;
      else
        denom = a - 2*b + c;
        if numer >= denom
          s = 1;
          t = 0;
          sqrDistance = a + 2*d + f;
        else
          s = numer/denom;
          t = 1-s;
          sqrDistance = s*(a*s + b*t + 2*d) ...
                      + t*(b*s + c*t + 2*e) + f;
        end
      end %of region 1
    end
  end
end

% account for numerical round-off error
if (sqrDistance < 0)
  sqrDistance = 0;
end

dist = sqrt(sqrDistance);

if nargout>1
  PP0 = B + s*E0 + t*E1;
end

end

















% Function for fast computation of the shortest distance between two line segments
%
% Algorithm implemented:
%   Vladimir J. LUMELSKY,
%   ``ON FAST COMPUTATION OF DISTANCE BETWEEN LINE SEGMENTS'',
%   Information Processing Letters 21 (1985) 55-61
%
%
% Input: ([start point of line1], [end point of line1], [start point of
% line2], [end point of line2])
%
% Output:   dist - shortest distance between the line segments (in N dimensions)
%           points (optional) - shortest points on the line segments
%
% Example:
% >> [dist,points] = distLinSeg([0 0], [1 1], [1 0], [2 0])
% >> dist = 0.7071
% >> points = [0.5 0.5; 1 0]
%
%
% 1.2.2015     - created: Ondrej Sluciak (osluciak@gmail.com)
%
function [dist,varargout] = distLinSeg(point1s,point1e,point2s,point2e)

d1  = point1e - point1s;
d2  = point2e - point2s;
d12 = point2s - point1s;

D1  = d1*d1';    %D1 = sum(d1.^2);
D2  = d2*d2';    %D2 = sum(d2.^2);

S1  = d1*d12';   % S1 = sum(d1.*d12);
S2  = d2*d12';   % S2 = sum(d2.*d12);
R   = d1*d2';    % R = sum(d1.*d2);

den = D1*D2-R^2;    %denominator

if (D1 == 0 || D2 == 0)     % if one of the segments is a point
    if (D1 ~= 0)            % if line1 is a segment and line2 is a point
        u = 0;
        t = S1/D1;

        t = fixbound(t);
 
    elseif (D2 ~= 0)        % if line2 is a segment and line 1 is a point
        t = 0;
        u = -S2/D2;

        u = fixbound(u);
  
    else                    % both segments are points
        t = 0;          
        u = 0;
    end
elseif (den == 0)           % if lines are parallel
    t = 0;
    u = -S2/D2;
    
    uf = fixbound(u);
    
    if (uf~= u)
        t = (uf*R+S1)/D1;
        t = fixbound(t);
    
        u = uf;
    end
else                        % general case
    
    t = (S1*D2-S2*R)/den;
    
    t = fixbound(t);
    
    u = (t*R-S2)/D2;
    uf = fixbound(u);
    
    if (uf ~= u)
        t = (uf*R+S1)/D1;
        t = fixbound(t);
      
        u = uf;
    end
end

% Compute distance given parameters 't' and 'u'
dist = norm(d1*t-d2*u-d12);   %dist = sqrt(sum((d1*t-d2*u-d12).^2));

if (nargout > 1)
    varargout = {[point1s + d1*t;point2s+d2*u]};
end

end
    
function num = fixbound(num)    % if num is out of (0,1) round to {0,1}

if (num < 0)
    num = 0;
elseif (num > 1)
    num = 1;
end

end
